simulink model "Lab6_PartB"  (R2025b)
settings: Solver=VariableStepAuto  StartTime=0.0  StopTime=1500  RelTol=1e-12
InitFcn:
  | Di = 30; % Tank inside diameter [cm]
  | Do = 1; % Out flow orifice diameter [cm]
  | A = pi*Di^2/4; % Area of the Tank [cm^2]
  | Ao = pi*Do^2/4; % Outlet area of Tank [cm^2]
  | g = 981; % Gravitational acceleration [cm/s^2]
  | Kp = 10; % Pump flow constant [cm^3/V.s]
undefined symbols (not defined in the file or in its folder): K, T
settings Model: Creator=Murl0  LastModifiedBy=Murl0

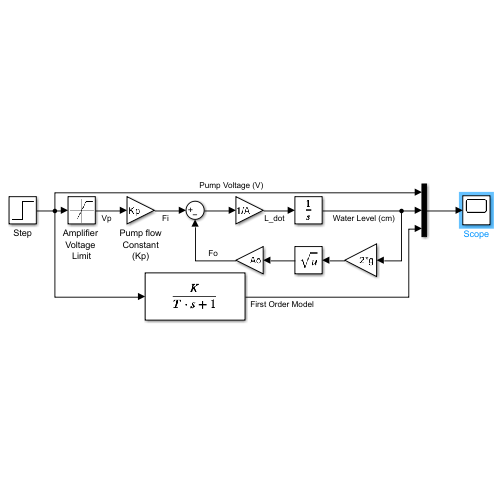
[thumbnail: Simulink's stored preview of the top-level diagram]
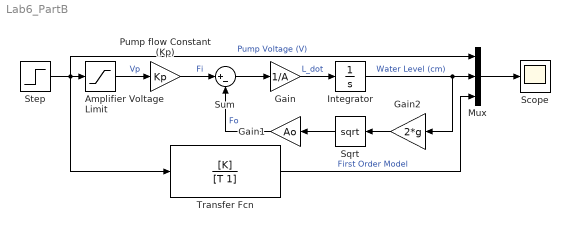
== system Lab6_PartB ==
  Amplifier Voltage Limit : Saturate  UpperLimit=50  LowerLimit=0
  Gain : Gain  Gain=1/A
  Gain1 : Gain  Gain=Ao
  Gain2 : Gain  Gain=2*g
  Integrator : Integrator
  Mux : Mux  Inputs=3
  Pump flow Constant (Kp) : Gain  Gain=Kp
  Scope : Scope
      settings: ActiveDisplayYMinimum=-3.3444238852727648  ActiveDisplayYMaximum=30.09981496745489
  Sqrt : Sqrt
  Step : Step  Time=0  After=18  SampleTime=0
  Sum : Sum  Inputs=|+-
  Transfer Fcn : TransferFcn  Numerator=[K]  Denominator=[T 1]
  wires:
  Step/1 -> Mux/1, Amplifier Voltage Limit/1, Transfer Fcn/1  "Pump Voltage (V)"
  Amplifier Voltage Limit/1 -> Pump flow Constant (Kp)/1  "Vp"
  Pump flow Constant (Kp)/1 -> Sum/1  "Fi"
  Sum/1 -> Gain/1
  Gain/1 -> Integrator/1  "L_dot"
  Integrator/1 -> Gain2/1, Mux/2  "Water Level (cm)"
  Mux/1 -> Scope/1
  Gain1/1 -> Sum/2  "Fo"
  Sqrt/1 -> Gain1/1
  Gain2/1 -> Sqrt/1
  Transfer Fcn/1 -> Mux/3  "First Order Model"
